simulink model "ScalerCalculator"  (R2021a)
settings: Solver=FixedStepDiscrete  StartTime=0.0  StopTime=10.0  RelTol=1e-3  EnableMultiTasking=on
libraries: simulink x3
settings Model: Creator=Momen El Sayed  LastModifiedBy=Momen El Sayed
settings DataIOCC: ReturnWorkspaceOutputs=off
settings OptimizationCC: DefaultParameterBehavior=Inlined  InlineInvariantSignals=on  EnableMemcpy=off  LifeSpan=1  EfficientTunableParamExpr=on
settings DebuggingCC: UnderspecifiedInitializationDetection=Classic  MergeDetectMultiDrivingBlocksExec=none  SFMachineParentedDataDiag=warning  ArithmeticOperatorsInVariantConditions=warning
settings ModelReferenceCC: PropagateSignalLabelsOutOfModel=off
settings SFSimCC: MATLABDynamicMemAlloc=off  CustomCodeUndefinedFunction=UseInterfaceOnly
settings RTWCC: SystemTargetFile=ert.tlc  GenCodeOnly=on  TemplateMakefile=ert_default_tmf  GenerateReport=on  IncludeHyperlinkInReport=on  LaunchReport=on  GenerateTraceInfo=on  GenerateTraceReport=on  GenerateTraceReportSl=on  GenerateTraceReportSf=on  GenerateTraceReportEml=on
settings CodeAppCC: ForceParamTrailComments=on  IgnoreCustomStorageClasses=off  OperatorAnnotations=on  SimulinkDataObjDesc=on  SFDataObjDesc=on  MATLABFcnDesc=on  InsertBlockDesc=on  StateflowObjectComments=on  MATLABSourceComments=on
settings ERTTargetCC: MultiwordLength=2048  GenerateSampleERTMain=on  InlinedParameterPlacement=NonHierarchical  ERTCustomFileTemplate=example_file_process.tlc

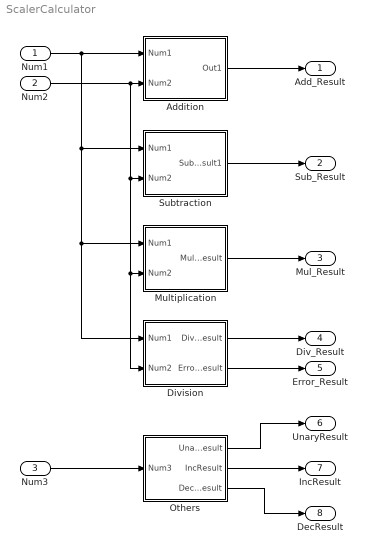
== system ScalerCalculator ==
  Num1 : Inport
  Num2 : Inport  Port=2
  Num3 : Inport  Port=3
  Addition : Subsystem  TreatAsAtomicUnit=on
      settings: RTWFcnNameOpts=Use subsystem name  RTWFileNameOpts=Use subsystem name
  Division : Subsystem  TreatAsAtomicUnit=on
      settings: RTWSystemCode=Nonreusable function  RTWFcnNameOpts=Use subsystem name  RTWFileNameOpts=Use subsystem name
  Multiplication : Subsystem  TreatAsAtomicUnit=on
      settings: RTWFcnNameOpts=Use subsystem name  RTWFileNameOpts=Use subsystem name
  Others : Subsystem
  Subtraction : Subsystem  TreatAsAtomicUnit=on
      settings: RTWFcnNameOpts=Use subsystem name  RTWFileNameOpts=Use subsystem name
  Add_Result : Outport
  Sub_Result : Outport  Port=2
  Mul_Result : Outport  Port=3
  Div_Result : Outport  Port=4
  Error_Result : Outport  Port=5
  UnaryResult : Outport  Port=6
  IncResult : Outport  Port=7
  DecResult : Outport  Port=8
  wires:
  Num2/1 -> Division/2(Num2), Multiplication/2(Num2), Subtraction/2(Num2), Addition/2(Num2)
  Addition/1(Out1) -> Add_Result/1
  Num1/1 -> Division/1(Num1), Multiplication/1(Num1), Subtraction/1(Num1), Addition/1(Num1)
  Subtraction/1(Sub_Result1) -> Sub_Result/1
  Multiplication/1(Mul_Result) -> Mul_Result/1
  Division/2(Error_Result) -> Error_Result/1
  Division/1(Div_Result) -> Div_Result/1
  Others/1(UnaryResult) -> UnaryResult/1
  Others/2(IncResult) -> IncResult/1
  Others/3(DecResult) -> DecResult/1
  Num3/1 -> Others/1(Num3)

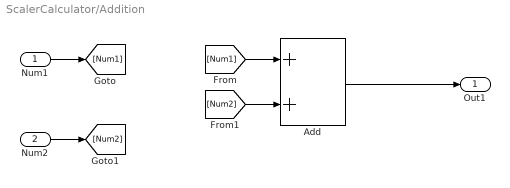
== system ScalerCalculator/Addition ==
  Num1 : Inport
  Num2 : Inport  Port=2
  Add : Sum
  Out1 : Outport
  wires:
  [Num2] -> Add/2
  Num1/1 -> [Num1]
  [Num1] -> Add/1
  Add/1 -> Out1/1
  Num2/1 -> [Num2]

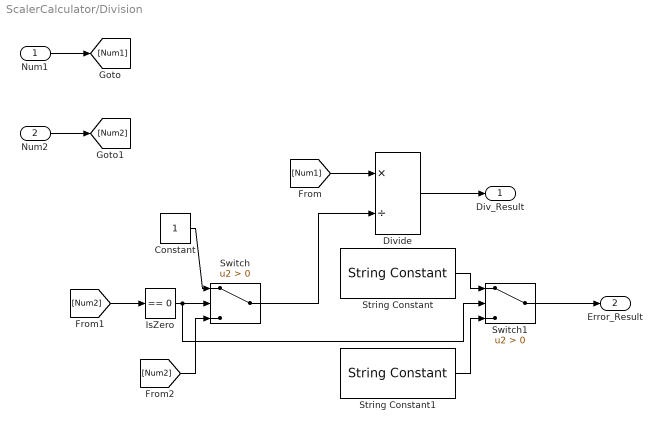
== system ScalerCalculator/Division ==
  Num1 : Inport
  Num2 : Inport  Port=2
  Constant : Constant
  Divide : Product  Inputs=*/
  IsZero : simulink/Logic and Bit Operations/Compare To Zero  relop===  OutDataTypeStr=boolean
  String Constant : StringConstant  String="\"Cann't Divide by Zero\""
  String Constant1 : StringConstant  String="\"No Problem\""
  Switch : Switch  Criteria=u2 > Threshold
  Switch1 : Switch  Criteria=u2 > Threshold
  Div_Result : Outport
  Error_Result : Outport  Port=2
  wires:
  [Num1] -> Divide/1
  Num2/1 -> [Num2]
  Num1/1 -> [Num1]
  [Num2] -> IsZero/1
  Divide/1 -> Div_Result/1
  IsZero/1 -> Switch1/2, Switch/2
  Constant/1 -> Switch/1
  [Num2] -> Switch/3
  Switch/1 -> Divide/2
  String Constant/1 -> Switch1/1
  String Constant1/1 -> Switch1/3
  Switch1/1 -> Error_Result/1

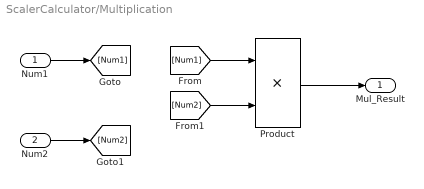
== system ScalerCalculator/Multiplication ==
  Num1 : Inport
  Num2 : Inport  Port=2
  Product : Product
  Mul_Result : Outport
  wires:
  [Num1] -> Product/1
  Num2/1 -> [Num2]
  Num1/1 -> [Num1]
  [Num2] -> Product/2
  Product/1 -> Mul_Result/1

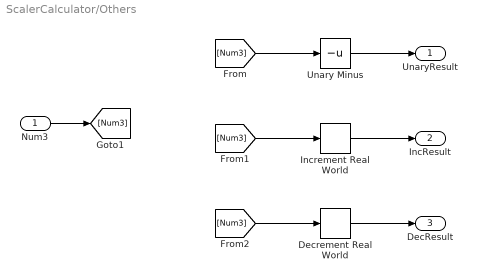
== system ScalerCalculator/Others ==
  Num3 : Inport
  Decrement Real World : simulink/Additional Math & Discrete/Additional Math: Increment - Decrement/Decrement Real World
      settings: SourceProductBaseCode=SL
  Increment Real World : simulink/Additional Math & Discrete/Additional Math: Increment - Decrement/Increment Real World
      settings: SourceProductBaseCode=SL
  Unary Minus : UnaryMinus
  UnaryResult : Outport
  IncResult : Outport  Port=2
  DecResult : Outport  Port=3
  wires:
  Num3/1 -> [Num3]
  [Num3] -> Unary Minus/1
  [Num3] -> Increment Real World/1
  [Num3] -> Decrement Real World/1
  Unary Minus/1 -> UnaryResult/1
  Increment Real World/1 -> IncResult/1
  Decrement Real World/1 -> DecResult/1

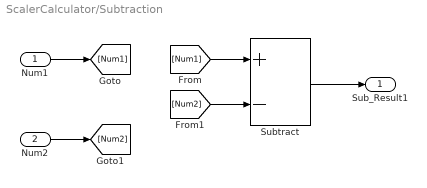
== system ScalerCalculator/Subtraction ==
  Num1 : Inport
  Num2 : Inport  Port=2
  Subtract : Sum  Inputs=+-
  Sub_Result1 : Outport
  wires:
  [Num1] -> Subtract/1
  Subtract/1 -> Sub_Result1/1
  [Num2] -> Subtract/2
  Num2/1 -> [Num2]
  Num1/1 -> [Num1]
